simulink model "HSM_4p6U10_Encoders_v01_06022022_NEW_ECC_2019a"  (R2019a)
settings: Solver=ode1  StartTime=0.0  StopTime=inf  FixedStep=Ts  RelTol=1e-3  EnableMultiTasking=on
values from neighbouring files (symbols this model uses):
  cold_low_offset = OLC*(2^26-1)    (= 64536.7492787)    [Parameters_4p6U10.m]
  cold_stroke = (OLC-OHC)*(2^26-1)    (= 50975.9994303)    [Parameters_4p6U10.m]
  hot_low_offset = OLH*(2^26-1)    (= 11504.7498714)    [Parameters_4p6U10.m]
  hot_stroke = (OHH-OLH)*(2^26-1)    (= 50961.9994305)    [Parameters_4p6U10.m]
undefined symbols (not defined in the file or in its folder): delayOnStart, read_BISSC_encoders
libraries: idelinklib_common x3, c280xlib x2, c2837xDlib x2
settings Model: ExtModeTrigDuration=8  Creator=vchilapu  LastModifiedBy=ThermoLift
settings DataIOCC: ReturnWorkspaceOutputs=off
settings OptimizationCC: DefaultUnderspecifiedDataType=single  EnhancedBackFolding=on  PassReuseOutputArgsAs=Individual arguments  MaxStackSize=512  OptimizeBlockOrder=speed
settings DebuggingCC: ParameterTunabilityLossMsg=error  ArithmeticOperatorsInVariantConditions=warning
settings HardwareCC: ProdBitPerChar=16  ProdBitPerInt=16  ProdBitPerPointer=32  ProdBitPerSizeT=32  ProdBitPerPtrDiffT=32  ProdLargestAtomicInteger=Integer  ProdLargestAtomicFloat=None  ProdWordSize=16  ProdLongLongMode=on  ProdHWDeviceType=Texas Instruments->C2000
settings SFSimCC: SimUserIncludeDirs=C:\Users\dzink\Desktop\NewFirmware  SimParseCustomCode=off  MATLABDynamicMemAlloc=off
settings SFSimCC: SimCustomHeaderCode=|
  | #include "memReadBISSC.h"
  | #include "delay_on_start.h"
  | #include "spi_lib_encoders.h"
  | #include "memReadSSI.h"
settings SFSimCC: SimUserSources=|
  | memReadBISSC.c
  | delay_on_start.c
  | spi_lib_encoders.c
  | memReadSSI.c
settings RTWCC: SystemTargetFile=ert.tlc  HardwareBoard=TI Delfino F28379D LaunchPad  TLCOptions=-aInlineSetEventsForThisBaseRateFcn=TLC_FALSE -aSuppressMultiTaskScheduler=TLC_FALSE -aRateBasedStepFcn=1  TemplateMakefile=ert_default_tmf  GenerateReport=on  RTWUseSimCustomCode=on  CustomInclude=C:\Users\dzink\Desktop\NewFirmware  Toolchain=Texas Instruments Code Composer Studio (C2000)  IncludeHyperlinkInReport=on  LaunchReport=on  GenerateTraceInfo=on  GenerateTraceReport=on  GenerateTraceReportSl=on  GenerateTraceReportSf=on  GenerateTraceReportEml=on
settings RTWCC: CustomHeaderCode=|
  | #include "memReadBISSC.h"
  | #include "delay_on_start.h"
  | #include "spi_lib_encoders.h"
  | #include "memReadSSI.h"
settings RTWCC: CustomSource=|
  | memReadBISSC.c
  | delay_on_start.c
  | spi_lib_encoders.c
  | memReadSSI.c
settings CodeAppCC: ForceParamTrailComments=on  IgnoreCustomStorageClasses=off  OperatorAnnotations=on  SimulinkDataObjDesc=on  SFDataObjDesc=on  InsertBlockDesc=on  StateflowObjectComments=on
settings ERTTargetCC: CodeReplacementLibrary=TI C28x  SupportContinuousTime=on  SupportNonInlinedSFcns=on

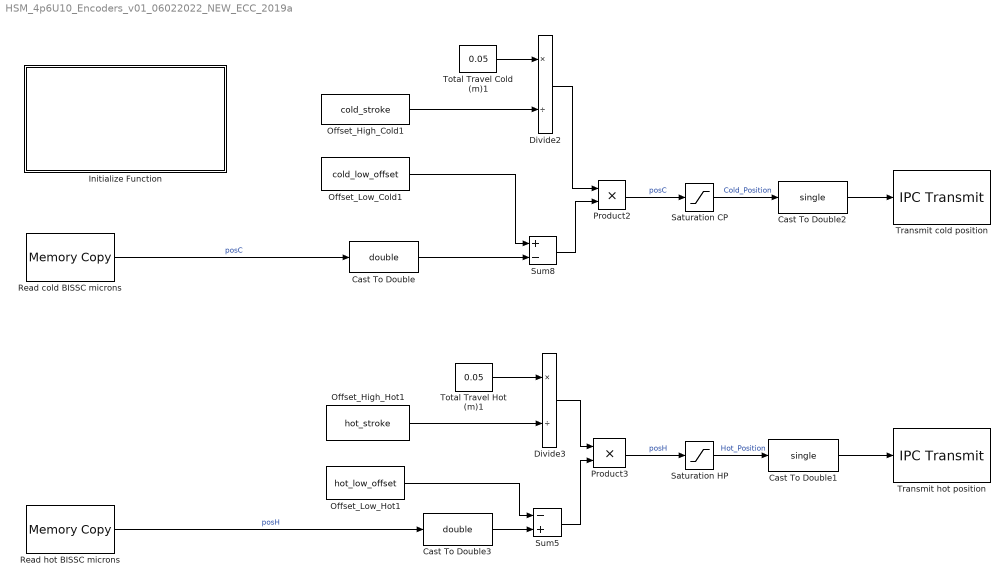
== system HSM_4p6U10_Encoders_v01_06022022_NEW_ECC_2019a ==
  Cast To Double : DataTypeConversion  OutDataTypeStr=double
  Cast To Double1 : DataTypeConversion  OutDataTypeStr=single
  Cast To Double2 : DataTypeConversion  OutDataTypeStr=single
  Cast To Double3 : DataTypeConversion  OutDataTypeStr=double
  Divide2 : Product  Inputs=*/
  Divide3 : Product  Inputs=*/
  Initialize Function : Subsystem  TreatAsAtomicUnit=on
  Offset_High_Cold1 : Constant  Value=cold_stroke
  Offset_High_Hot1 : Constant  Value=hot_stroke
  Offset_Low_Cold1 : Constant  Value=cold_low_offset
  Offset_Low_Hot1 : Constant  Value=hot_low_offset
  Product2 : Product
  Product3 : Product
  Read cold BISSC microns : idelinklib_common/Memory Copy  copyFrom=Specified source code symbol  copyFromAddressSource=Specify via dialog  copyFromAddress=hex2dec('00001000')  copyFromSrcCode=&cold_encoder_pos  dataTypeFrom=uint32  dataDimensionFrom=1  useOffsetFrom=off  offsetFromSrc=Specify via dialog  offsetFrom=0  strideFrom=1  copyTo=Output port  copyToAddressSource=Specify via dialog  copyToAddress=hex2dec('00002000')  copyToSrcCode=myVariableDst  dataTypeTo=uint32  useOffsetTo=off  offsetToSrc=Specify via dialog  offsetTo=0  strideTo=1  sampleTime=Ts  useInitValue=off  initValueSrc=Specify constant value  initValue=1  initValueSrcCode=myInitValueVariable  useAsMask=off  maskOperator=bitwise AND  useTermValue=off  termValue=1  isRealtimeEnabled=off  emitCCBeforeWrite=on  CCBeforeWrite=read_BISSC_encoders();  emitCCAfterWrite=off  CCAfterWrite=/* Custom Code After Write*/  useDMACopy=off  enableBlockingMode=off
      settings: SourceProductName=MATLAB Coder  SourceProductBaseCode=ME
  Read hot BISSC microns : idelinklib_common/Memory Copy  copyFrom=Specified source code symbol  copyFromAddressSource=Specify via dialog  copyFromAddress=hex2dec('00001000')  copyFromSrcCode=&hot_encoder_pos  dataTypeFrom=uint32  dataDimensionFrom=1  useOffsetFrom=off  offsetFromSrc=Specify via dialog  offsetFrom=0  strideFrom=1  copyTo=Output port  copyToAddressSource=Specify via dialog  copyToAddress=hex2dec('00002000')  copyToSrcCode=myVariableDst  dataTypeTo=uint32  useOffsetTo=off  offsetToSrc=Specify via dialog  offsetTo=0  strideTo=1  sampleTime=Ts  useInitValue=off  initValueSrc=Specify constant value  initValue=1  initValueSrcCode=myInitValueVariable  useAsMask=off  maskOperator=bitwise AND  useTermValue=off  termValue=1  isRealtimeEnabled=off  emitCCBeforeWrite=off  CCBeforeWrite=/* Custom Code Before Write*/  emitCCAfterWrite=off  CCAfterWrite=/* Custom Code After Write*/  useDMACopy=off  enableBlockingMode=off
      settings: SourceProductName=MATLAB Coder  SourceProductBaseCode=ME
  Saturation CP : Saturate  UpperLimit=0.050  LowerLimit=0.000  OutMin=[0]  OutMax=[0.050]
  Saturation HP : Saturate  UpperLimit=0.050  LowerLimit=0.000  OutMin=[0]  OutMax=[0.050]
  Sum5 : Sum  Inputs=-+
  Sum8 : Sum  Inputs=+-
  Total Travel Cold (m)1 : Constant  Value=0.05
  Total Travel Hot (m)1 : Constant  Value=0.05
  Transmit cold position : c2837xDlib/IPC Transmit  SelectChannel=0  EnableBlocking=off
      settings: SourceProductName=Embedded Coder Support Package for Texas Instruments C2000 Processors  SourceProductBaseCode=TIC2000
  Transmit hot position : c2837xDlib/IPC Transmit  SelectChannel=1  EnableBlocking=off
      settings: SourceProductName=Embedded Coder Support Package for Texas Instruments C2000 Processors  SourceProductBaseCode=TIC2000
  wires:
  Read hot BISSC microns/1 -> Cast To Double3/1  "posH"
  Read cold BISSC microns/1 -> Cast To Double/1  "posC"
  Offset_Low_Hot1/1 -> Sum5/1
  Offset_High_Hot1/1 -> Divide3/2
  Divide2/1 -> Product2/1
  Offset_High_Cold1/1 -> Divide2/2
  Total Travel Hot (m)1/1 -> Divide3/1
  Sum8/1 -> Product2/2
  Cast To Double/1 -> Sum8/2
  Offset_Low_Cold1/1 -> Sum8/1
  Total Travel Cold (m)1/1 -> Divide2/1
  Divide3/1 -> Product3/1
  Sum5/1 -> Product3/2
  Cast To Double3/1 -> Sum5/2
  Saturation CP/1 -> Cast To Double2/1  "Cold_Position"
  Saturation HP/1 -> Cast To Double1/1  "Hot_Position"
  Product2/1 -> Saturation CP/1  "posC"
  Product3/1 -> Saturation HP/1  "posH"
  Cast To Double2/1 -> Transmit cold position/1
  Cast To Double1/1 -> Transmit hot position/1

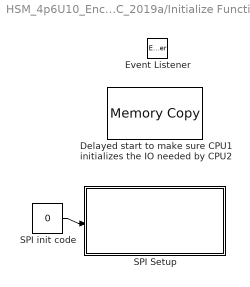
== system HSM_4p6U10_Encoders_v01_06022022_NEW_ECC_2019a/Initialize Function ==
  Delayed start to make sure CPU1 initializes the IO needed by CPU2 : idelinklib_common/Memory Copy  copyFrom=Specified source code symbol  copyFromAddressSource=Specify via dialog  copyFromAddress=hex2dec('00001000')  copyFromSrcCode=&delayDummy  dataTypeFrom=uint32  dataDimensionFrom=1  useOffsetFrom=off  offsetFromSrc=Specify via dialog  offsetFrom=0  strideFrom=1  copyTo=Specified source code symbol  copyToAddressSource=Specify via dialog  copyToAddress=hex2dec('00002000')  copyToSrcCode=&delayDummy  dataTypeTo=uint32  useOffsetTo=off  offsetToSrc=Specify via dialog  offsetTo=0  strideTo=1  sampleTime=inf  useInitValue=on  initValueSrc=Specify constant value  initValue=1  initValueSrcCode=myInitValueVariable  useAsMask=off  maskOperator=bitwise AND  useTermValue=off  termValue=1  isRealtimeEnabled=on  emitCCBeforeWrite=on  CCBeforeWrite=delayOnStart();  emitCCAfterWrite=off  CCAfterWrite=/* Custom Code After Write*/  useDMACopy=off  enableBlockingMode=off
      settings: SourceProductName=MATLAB Coder  SourceProductBaseCode=ME
  Event Listener : EventListener  DisableCoverage=on  EventName=reset
  SPI Setup : Subsystem  TreatAsAtomicUnit=on
  SPI init code : Constant  Value=0  OutDataTypeStr=uint16
  wires:
  SPI init code/1 -> SPI Setup/Enable

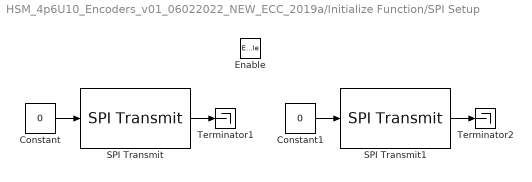
== system HSM_4p6U10_Encoders_v01_06022022_NEW_ECC_2019a/Initialize Function/SPI Setup ==
  Enable : EnablePort
  Constant : Constant  Value=0  OutDataTypeStr=uint16  SampleTime=-1
  Constant1 : Constant  Value=0  OutDataTypeStr=uint16  SampleTime=-1
  SPI Transmit : c280xlib/SPI Transmit  SPISelect=SPI_A  ClockPolarity=Rising_edge  ClockPhase=No_delay  SPIModule=uint32(0)  Mode=Master  BusSpeed=uint32(1000000)  FirstBitToTransfer=Most significant bit (MSB)  ClockMode=0  BlockFunction=Write  EnableRegisterAddress=on  RegisterAddress=0  OutputDataType=int8  OutputDataLength=1  BlockingMode=off  DataBits=16  UseCustomSSPin=Provided by the SPI peripheral  ActiveLowSSPin=Active low  Pin=0
      settings: SourceProductName=Embedded Coder Support Package for Texas Instruments C2000 Processors  SourceProductBaseCode=TIC2000
  SPI Transmit1 : c280xlib/SPI Transmit  SPISelect=SPI_B  ClockPolarity=Rising_edge  ClockPhase=No_delay  SPIModule=uint32(0)  Mode=Master  BusSpeed=uint32(1000000)  FirstBitToTransfer=Most significant bit (MSB)  ClockMode=0  BlockFunction=Write  EnableRegisterAddress=on  RegisterAddress=0  OutputDataType=int8  OutputDataLength=1  BlockingMode=off  DataBits=16  UseCustomSSPin=Provided by the SPI peripheral  ActiveLowSSPin=Active low  Pin=0
      settings: SourceProductName=Embedded Coder Support Package for Texas Instruments C2000 Processors  SourceProductBaseCode=TIC2000
  Terminator1 : Terminator
  Terminator2 : Terminator
  wires:
  SPI Transmit/1 -> Terminator1/1
  SPI Transmit1/1 -> Terminator2/1
  Constant/1 -> SPI Transmit/1
  Constant1/1 -> SPI Transmit1/1
